simulink model "ModeloCorrigido_feedbackLinearizationMambo"  (R2021a)
settings: Solver=VariableStepAuto  StartTime=0  StopTime=60  FixedStep=4e-3  RelTol=1e-12
InitFcn:
  | init
undefined symbols (not defined in the file): a, b, c, Controller, Earth, g, init, J, Ki, rho, sigma, T, Ts, Vehicle, WGS84
libraries: pid_lib x8, sharedtransform x8, shared6dof x2, aerolibasang x2, aerolibtransform2 x2, dynamicsLibrary x1
(part 2 of 2)

== system ModeloCorrigido_feedbackLinearizationMambo/Mambo Model/AC model/Gravity Force Calculation ==
  DCMbe : Inport
  gravity : Inport  Port=2  Unit=m/s^2
  Gain1 : Gain  Gain=Vehicle.Airframe.mass
  Product : Product  Multiplication=Matrix(*)
  gravity force : Outport  Unit=N  VectorParamsAs1DForOutWhenUnconnected=off
  wires:
  gravity/1 -> Gain1/1
  Gain1/1 -> Product/2  "gravity force NED"
  Product/1 -> gravity force/1
  DCMbe/1 -> Product/1

== system ModeloCorrigido_feedbackLinearizationMambo/Mambo Model1/AC model/Applied Force Calculation ==
  gravity force : Inport  Unit=N
  Aerodynamic Forces : Inport  Port=2  Unit=N
  Motor Forces : Inport  Port=3  Unit=N
  Add1 : Sum  Inputs=+++
  Signal Specification : SignalSpecification  Dimensions=3
  External Forces : Outport  Unit=N  VectorParamsAs1DForOutWhenUnconnected=off
  wires:
  Add1/1 -> Signal Specification/1
  Motor Forces/1 -> Add1/3  "Motor Thrust"
  Aerodynamic Forces/1 -> Add1/2
  gravity force/1 -> Add1/1
  Signal Specification/1 -> External Forces/1

== system ModeloCorrigido_feedbackLinearizationMambo/Mambo Model1/AC model/Drag Calculation ==
  Density : Inport  Unit=kg/m^3
  Vb : Inport  Port=2  Unit=m/second
  Drag Calc : Subsystem
  Gain3 : Gain  Gain=-1
  Product : Product  RndMeth=Zero
  Sign : Signum  ZeroCross=off
  Drag : Outport  Unit=N  VectorParamsAs1DForOutWhenUnconnected=off
  wires:
  Density/1 -> Drag Calc/1(Density)
  Sign/1 -> Gain3/1
  Drag Calc/1(drag) -> Product/1
  Gain3/1 -> Product/2
  Product/1 -> Drag/1  "xDrag"
  Vb/1 -> Sign/1, Drag Calc/2(vel)

== system ModeloCorrigido_feedbackLinearizationMambo/Mambo Model1/AC model/Gravity Force Calculation ==
  DCMbe : Inport
  gravity : Inport  Port=2  Unit=m/s^2
  Gain1 : Gain  Gain=Vehicle.Airframe.mass
  Product : Product  Multiplication=Matrix(*)
  gravity force : Outport  Unit=N  VectorParamsAs1DForOutWhenUnconnected=off
  wires:
  gravity/1 -> Gain1/1
  Gain1/1 -> Product/2  "gravity force NED"
  Product/1 -> gravity force/1
  DCMbe/1 -> Product/1

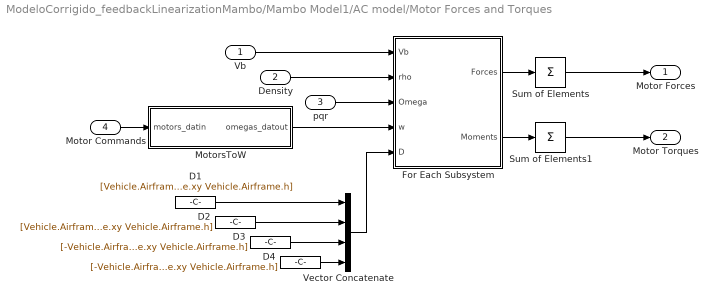
== system ModeloCorrigido_feedbackLinearizationMambo/Mambo Model1/AC model/Motor Forces and Torques ==
  Vb : Inport
  Density : Inport  Port=2
  pqr : Inport  Port=3
  Motor Commands : Inport  Port=4
  D1 : Constant  Value=[Vehicle.Airframe.xy -Vehicle.Airframe.xy Vehicle.Airframe.h]
  D2 : Constant  Value=[Vehicle.Airframe.xy Vehicle.Airframe.xy Vehicle.Airframe.h]
  D3 : Constant  Value=[-Vehicle.Airframe.xy Vehicle.Airframe.xy Vehicle.Airframe.h]
  D4 : Constant  Value=[-Vehicle.Airframe.xy -Vehicle.Airframe.xy Vehicle.Airframe.h]
  For Each Subsystem : Subsystem  TreatAsAtomicUnit=on
  MotorsToW : Subsystem
  Sum of Elements : Sum  Inputs=+  CollapseMode=Specified dimension  CollapseDim=2
  Sum of Elements1 : Sum  Inputs=+  CollapseMode=Specified dimension  CollapseDim=2
  Vector Concatenate : Concatenate  NumInputs=4  Mode=Multidimensional array  ConcatenateDimension=2
  Motor Forces : Outport  Unit=N  VectorParamsAs1DForOutWhenUnconnected=off
  Motor Torques : Outport  Port=2  Unit=N*m  VectorParamsAs1DForOutWhenUnconnected=off
  wires:
  D4/1 -> Vector Concatenate/4
  MotorsToW/1(omegas_datout) -> For Each Subsystem/4(w)
  Vector Concatenate/1 -> For Each Subsystem/5(D)
  For Each Subsystem/2(Moments) -> Sum of Elements1/1
  pqr/1 -> For Each Subsystem/3(Omega)
  Vb/1 -> For Each Subsystem/1(Vb)
  Motor Commands/1 -> MotorsToW/1(motors_datin)
  D1/1 -> Vector Concatenate/1
  D3/1 -> Vector Concatenate/3
  D2/1 -> Vector Concatenate/2
  Sum of Elements1/1 -> Motor Torques/1
  Density/1 -> For Each Subsystem/2(rho)
  Sum of Elements/1 -> Motor Forces/1
  For Each Subsystem/1(Forces) -> Sum of Elements/1

== system ModeloCorrigido_feedbackLinearizationMambo/Mambo Model/AC model/Drag Calculation/Drag Calc ==
  Density : Inport  Unit=kg/m^3
  vel : Inport  Port=2  Unit=m/s
  Dynamic Pressure : aerolibasang/Dynamic Pressure
  Gain : Gain  Gain=[.25 .25]
  Mux1 : Mux  Inputs=2
  Product : Product  Inputs=3  RndMeth=Zero
  diameter : Constant  Value=Vehicle.Airframe.diameter  SampleTime=0
  dragCoeff : Constant  Value=Vehicle.Airframe.Cdx  SampleTime=0
  drag : Outport  Unit=N  VectorParamsAs1DForOutWhenUnconnected=off
  wires:
  Product/1 -> drag/1
  dragCoeff/1 -> Product/3  "Cd"
  Dynamic Pressure/1 -> Product/1  "q"
  diameter/1 -> Gain/1, Mux1/2
  Mux1/1 -> Product/2  "S"
  Gain/1 -> Mux1/1
  vel/1 -> Dynamic Pressure/1
  Density/1 -> Dynamic Pressure/2

== system ModeloCorrigido_feedbackLinearizationMambo/Mambo Model1/AC model/Drag Calculation/Drag Calc ==
  Density : Inport  Unit=kg/m^3
  vel : Inport  Port=2  Unit=m/s
  Dynamic Pressure : aerolibasang/Dynamic Pressure
  Gain : Gain  Gain=[.25 .25]
  Mux1 : Mux  Inputs=2
  Product : Product  Inputs=3  RndMeth=Zero
  diameter : Constant  Value=Vehicle.Airframe.diameter  SampleTime=0
  dragCoeff : Constant  Value=Vehicle.Airframe.Cdx  SampleTime=0
  drag : Outport  Unit=N  VectorParamsAs1DForOutWhenUnconnected=off
  wires:
  Product/1 -> drag/1
  dragCoeff/1 -> Product/3  "Cd"
  Dynamic Pressure/1 -> Product/1  "q"
  diameter/1 -> Gain/1, Mux1/2
  Mux1/1 -> Product/2  "S"
  Gain/1 -> Mux1/1
  vel/1 -> Dynamic Pressure/1
  Density/1 -> Dynamic Pressure/2

== system ModeloCorrigido_feedbackLinearizationMambo/Mambo Model1/AC model/Motor Forces and Torques/For Each Subsystem ==
  Vb : Inport  PortDimensions=3
  rho : Inport  Port=2  PortDimensions=1
  Omega : Inport  Port=3
  w : Inport  Port=4  Partition=on  PartitionDimension=1  PartitionWidth=1  PartitionOffset=0
  D : Inport  Port=5  Partition=on  PartitionDimension=2  PartitionWidth=1  PartitionOffset=0
  For Each : ForEach  DisableCoverage=on
  Rotor Dynamics : dynamicsLibrary/Rotor Dynamics  SystemSampleTime=-1  VariantActivationTime=update diagram  Latency=0  AutoFrameSizeCalculation=off
  Forces : Outport  ConcatenationDimension=2  VectorParamsAs1DForOutWhenUnconnected=off
  Moments : Outport  Port=2  ConcatenationDimension=2  VectorParamsAs1DForOutWhenUnconnected=off
  wires:
  Rotor Dynamics/1 -> Forces/1
  Rotor Dynamics/2 -> Moments/1
  Vb/1 -> Rotor Dynamics/1
  Omega/1 -> Rotor Dynamics/2
  rho/1 -> Rotor Dynamics/3
  D/1 -> Rotor Dynamics/5
  w/1 -> Rotor Dynamics/4

== system ModeloCorrigido_feedbackLinearizationMambo/Mambo Model1/AC model/Motor Forces and Torques/MotorsToW ==
  motors_datin : Inport
  Motordirections : Gain  Gain=[1 -1 1 -1]  ParamDataTypeStr=single  OutDataTypeStr=Inherit: Inherit via back propagation  SaturateOnIntegerOverflow=on
  Motordirections1 : Gain  Gain=[1 -1 1 -1]  ParamDataTypeStr=single  OutDataTypeStr=Inherit: Inherit via back propagation  SaturateOnIntegerOverflow=on
  Saturation5 : Saturate  UpperLimit=Vehicle.Motor.maxLimit  LowerLimit=Vehicle.Motor.minLimit  OutDataTypeStr=Inherit: Inherit via back propagation
  Signed Sqrt : Sqrt  Operator=signedSqrt  OutDataTypeStr=Inherit: Inherit via back propagation  SaturateOnIntegerOverflow=on
  motorsToW2_Gain : Gain  Gain=Vehicle.Motor.commandToW2Gain  ParamDataTypeStr=single  OutDataTypeStr=Inherit: Inherit via back propagation  SaturateOnIntegerOverflow=on
  omegas_datout : Outport  VectorParamsAs1DForOutWhenUnconnected=off
  wires:
  motorsToW2_Gain/1 -> Signed Sqrt/1
  Motordirections/1 -> Saturation5/1
  Saturation5/1 -> Motordirections1/1
  Motordirections1/1 -> motorsToW2_Gain/1
  Signed Sqrt/1 -> omegas_datout/1
  motors_datin/1 -> Motordirections/1

== matlab function ModeloCorrigido_feedbackLinearizationMambo/ 1 ==
  data: quart input; e input; w input size=4; m output; v input; n output; o output; sigma parameter; linearVel input; J parameter; k output; g parameter
function [m, n, o, k] = feedbackLin(quart,e, w, v, sigma,linearVel, J,g)

ml = w(1);
nl = w(2);
ol = w(3);
kl = w(4);

q0 = quart(1);
q1 = quart(2);
q2 = quart(3);
q3 = quart(4);

p = v(1);
q = v(2);
r = v(3);

Jx = J(1);
Jy = J(2);
Jz = J(3);

vy = linearVel(2);
vx = linearVel(1);

A = [ q0 + q1^2/q0,  q3 + q1*q2/q0,  -q2 + q1*q3/q0;
      -q3 + q1*q2/q0,  q0 + q2^2/q0,   q1 + q2*q3/q0;
      q2 + q1*q3/q0,  -q1 + q2*q3/q0,  q0 + q3^2/q0];
  
dq0 = 1/2*(-q1*p - q2*q - q3*r);
dq1 = 1/2*(q0*p - q3*q + q2*r);
dq2 = 1/2*(q3*p + q0*q - q1*r);
dq3 = 1/2*(-q2*p + q1*q + q0*r);

dp = (Jy-Jz)/Jx*q*r;
dq = (Jz-Jx)/Jy*p*r;
dr = (Jx-Jy)/Jz*q*p;

SigmaQ1 = sigma(1);
SigmaQ2 = sigma(2);
SigmaQ3 = sigma(3);
SigmaZ = sigma(4);

B = [(2*ml - (dq0*p - dq3*q + dq2*r) - (q0*dp-q3*dq+q2*dr))/SigmaQ1;
     (2*nl - (dq3*p + dq0*q - dq1*r) - (q3*dp+q0*dq-q1*dr))/SigmaQ2;
     (2*ol - (-dq2*p + dq3*q + dq0*r) - (-q2*dp+q1*dq+q0*dr))/SigmaQ3];
 
C = A*B;

phi = e(1);
theta = e(2);

m = C(1);
n = C(2);
o = C(3);
k = (kl-g)/(SigmaZ*cos(phi)*cos(theta));

== matlab function ModeloCorrigido_feedbackLinearizationMambo/ 2 ==
  data: quart input; e input; w input size=4; m output; v input; n output; o output; sigma parameter; linearVel input; J parameter; k output; g parameter
function [m, n, o, k] = feedbackLin(quart,e, w, v, sigma,linearVel, J,g)

ml = w(1);
nl = w(2);
ol = w(3);
kl = w(4);

q0 = quart(1);
q1 = quart(2);
q2 = quart(3);
q3 = quart(4);

p = v(1);
q = v(2);
r = v(3);

Jx = J(1);
Jy = J(2);
Jz = J(3);

vy = linearVel(2);
vx = linearVel(1);

A = [ q0 + q1^2/q0,  q3 + q1*q2/q0,  -q2 + q1*q3/q0;
      -q3 + q1*q2/q0,  q0 + q2^2/q0,   q1 + q2*q3/q0;
      q2 + q1*q3/q0,  -q1 + q2*q3/q0,  q0 + q3^2/q0];
  
dq0 = 1/2*(-q1*p - q2*q - q3*r);
dq1 = 1/2*(q0*p - q3*q + q2*r);
dq2 = 1/2*(q3*p + q0*q - q1*r);
dq3 = 1/2*(-q2*p + q1*q + q0*r);

dp = (Jy-Jz)/Jx*q*r;
dq = (Jz-Jx)/Jy*p*r;
dr = (Jx-Jy)/Jz*q*p;

SigmaQ1 = sigma(1);
SigmaQ2 = sigma(2);
SigmaQ3 = sigma(3);
SigmaZ = sigma(4);

B = [(2*ml - (dq0*p - dq3*q + dq2*r) - (q0*dp-q3*dq+q2*dr))/SigmaQ1;
     (2*nl - (dq3*p + dq0*q - dq1*r) - (q3*dp+q0*dq-q1*dr))/SigmaQ2;
     (2*ol - (-dq2*p + dq3*q + dq0*r) - (-q2*dp+q1*dq+q0*dr))/SigmaQ3];
 
C = A*B;

phi = e(1);
theta = e(2);

m = C(1);
n = C(2);
o = C(3);
k = (kl-g)/(SigmaZ*cos(phi)*cos(theta));

== matlab function ModeloCorrigido_feedbackLinearizationMambo/Mambo Model/AC model/rotMatrix ==
  data: eul input size=[1,3]; rotm output size=[3,3]
function rotm = rotMat(eul)

rotm = eul2rotm(eul);
